simulink model "SistemSaKlipom"  (R2015b)
settings: Solver=VariableStepAuto  StartTime=0.0  StopTime=10.0  RelTol=1e-3
values from neighbouring files (symbols this model uses):
  C1 = [1 0 0 0]    [Parametri.m]
undefined symbols (not defined in the file or in its folder): C2, D1, D2, D3, J1, J2, J3
libraries: powerlib_meascontrol x1
settings Model: Creator=user  LastModifiedBy=user

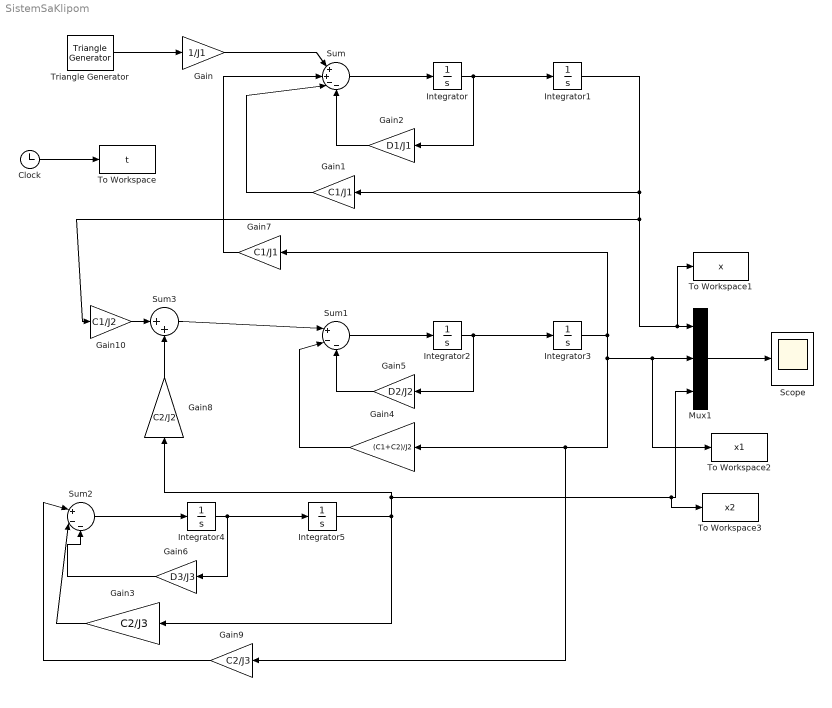
== system SistemSaKlipom ==
  Clock : Clock
  Gain : Gain  Gain=1/J1
  Gain1 : Gain  Gain=C1/J1
  Gain10 : Gain  Gain=C1/J2
  Gain2 : Gain  Gain=D1/J1
  Gain3 : Gain  Gain=C2/J3
  Gain4 : Gain  Gain=(C1+C2)/J2
  Gain5 : Gain  Gain=D2/J2
  Gain6 : Gain  Gain=D3/J3
  Gain7 : Gain  Gain=C1/J1
  Gain8 : Gain  Gain=C2/J2
  Gain9 : Gain  Gain=C2/J3
  Integrator{,1..5} (6 alike) : Integrator
  Mux1 : Mux  Inputs=3
  Scope : Scope
  Sum : Sum  Inputs=|++--
  Sum1 : Sum  Inputs=|+--
  Sum2 : Sum  Inputs=|+--
  Sum3 : Sum  Inputs=|++
  To Workspace : ToWorkspace  VariableName=t  SampleTime=-1
      settings: Save2DSignal=2-D array (concatenate along first dimension)
  To Workspace1 : ToWorkspace  VariableName=x  SampleTime=-1
      settings: Save2DSignal=2-D array (concatenate along first dimension)
  To Workspace2 : ToWorkspace  VariableName=x1  SampleTime=-1
      settings: Save2DSignal=2-D array (concatenate along first dimension)
  To Workspace3 : ToWorkspace  VariableName=x2  SampleTime=-1
      settings: Save2DSignal=2-D array (concatenate along first dimension)
  Triangle Generator : powerlib_meascontrol/Pulse & Signal Generators/Triangle Generator  Freq=1  Phase=90  Ts=0
  wires:
  Clock/1 -> To Workspace/1
  Gain/1 -> Sum/1
  Sum/1 -> Integrator/1
  Integrator/1 -> Gain2/1, Integrator1/1
  Gain2/1 -> Sum/4
  Gain1/1 -> Sum/3
  Sum1/1 -> Integrator2/1
  Integrator2/1 -> Integrator3/1, Gain5/1
  Gain5/1 -> Sum1/3
  Integrator3/1 -> Gain9/1, Gain4/1, To Workspace2/1, Mux1/2, Gain7/1
  Sum2/1 -> Integrator4/1
  Integrator4/1 -> Gain6/1, Integrator5/1
  Gain6/1 -> Sum2/3
  Gain4/1 -> Sum1/2
  Gain7/1 -> Sum/2
  Gain3/1 -> Sum2/2
  Gain9/1 -> Sum2/1
  Integrator5/1 -> To Workspace3/1, Mux1/3, Gain8/1, Gain3/1
  Mux1/1 -> Scope/1
  Triangle Generator/1 -> Gain/1
  Gain8/1 -> Sum3/2
  Gain10/1 -> Sum3/1
  Integrator1/1 -> To Workspace1/1, Mux1/1, Gain10/1, Gain1/1
  Sum3/1 -> Sum1/1
